simulink model "three_phase_diode_rectifier_updated"  (R2025a)
settings: Solver=VariableStepAuto  StartTime=0.0  StopTime=0.5  RelTol=1e-3
libraries: spsDiodeLib x6, spsACVoltageSourceLib x3, spsCurrentMeasurementLib x3, spsVoltageMeasurementLib x3, spsSeriesRLCBranchLib x2, spsMeanLib x1, spsTHDLib x1, spspowerguiLib x1
settings Model: Creator=yiğit  LastModifiedBy=yiğit

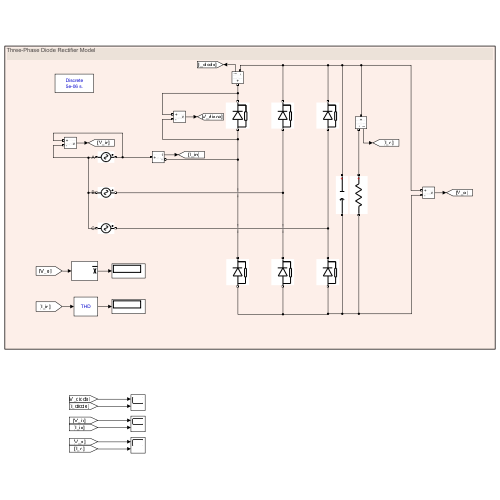
[thumbnail: Simulink's stored preview of the top-level diagram]
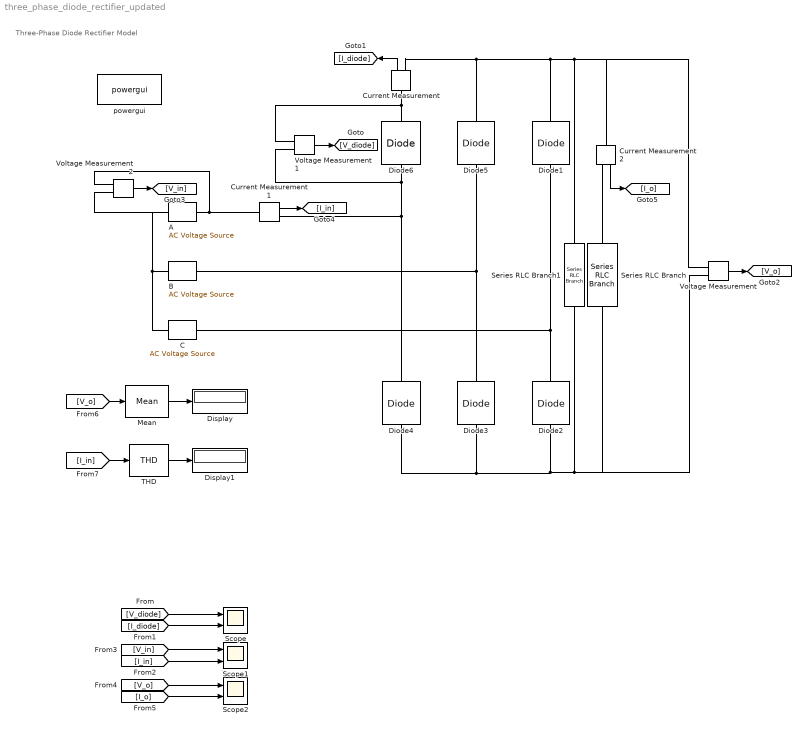
== system three_phase_diode_rectifier_updated ==
  note: Three-Phase Diode Rectifier Model
  A : spsACVoltageSourceLib/AC Voltage Source  Amplitude=136.082  Phase=0  Frequency=50  SampleTime=0  Measurements=None  BusType=swing  Pref=10e3  Qref=0  Qmin=-inf  Qmax=+inf
  B : spsACVoltageSourceLib/AC Voltage Source  Amplitude=136.082  Phase=120  Frequency=50  SampleTime=0  Measurements=None  BusType=swing  Pref=10e3  Qref=0  Qmin=-inf  Qmax=+inf
  C : spsACVoltageSourceLib/AC Voltage Source  Amplitude=136.082  Phase=240  Frequency=50  SampleTime=0  Measurements=None  BusType=swing  Pref=10e3  Qref=0  Qmin=-inf  Qmax=+inf
  Current Measurement : spsCurrentMeasurementLib/Current Measurement  PhasorSimulation=off  OutputType=Complex  PSBequivalent=0
  Current Measurement1 : spsCurrentMeasurementLib/Current Measurement  PhasorSimulation=off  OutputType=Complex  PSBequivalent=0
  Current Measurement2 : spsCurrentMeasurementLib/Current Measurement  PhasorSimulation=off  OutputType=Complex  PSBequivalent=0
  Diode{1..6} (6 alike) : spsDiodeLib/Diode  Ron=1e-3  Lon=0  Vf=0  IC=0  UseSnubber=0  Rs=1e6  Cs=1e-12  Measurements=off
  Display : Display
  Display1 : Display
  Mean : spsMeanLib/Mean  Freq=50  Vinit=0  Ts=0
  Scope : Scope  NumInputPorts=2
      settings: ActiveDisplayYMinimum=-34.164994069394211  ActiveDisplayYMaximum=260.46816184047532
  Scope1 : Scope  NumInputPorts=2
      settings: ActiveDisplayYMinimum=-170.10249999999996  ActiveDisplayYMaximum=170.10249999999996
  Scope2 : Scope  NumInputPorts=2
      settings: ActiveDisplayYMinimum=175.237742445763  ActiveDisplayYMaximum=464.02263493938636  DataLoggingVariableName=ScopeData2
  Series RLC Branch : spsSeriesRLCBranchLib/Series RLC Branch  LConnTagsString=__new0  RConnTagsString=__new0  BranchType=R  Resistance=25  Inductance=1e-3  SetiL0=off  InitialCurrent=0  Capacitance=1e-6  Setx0=off  InitialVoltage=0  Measurements=None
  Series RLC Branch1 : spsSeriesRLCBranchLib/Series RLC Branch  LConnTagsString=__new0  RConnTagsString=__new0  BranchType=C  Resistance=1  Inductance=1e-3  SetiL0=off  InitialCurrent=0  Capacitance=100e-6  Setx0=off  InitialVoltage=0  Measurements=None
  THD : spsTHDLib/THD  Freq=60  Ts=0
  Voltage Measurement : spsVoltageMeasurementLib/Voltage Measurement  PhasorSimulation=off  OutputType=Complex  PSBequivalent=0
  Voltage Measurement1 : spsVoltageMeasurementLib/Voltage Measurement  PhasorSimulation=off  OutputType=Complex  PSBequivalent=0
  Voltage Measurement2 : spsVoltageMeasurementLib/Voltage Measurement  PhasorSimulation=off  OutputType=Complex  PSBequivalent=0
  powergui : spspowerguiLib/powergui  Priority=1  SimulationMode=Discrete  SampleTime=5e-6  frequency=60  Iterations=50  frequencyindice=50  Pbase=100e6  ErrMax=1e-4  UnitsV=kV  UnitsW=MW  buscounter=0  FunctionMessages=off  echomessages=off  EnableUseOfTLC=off  CurrentSourceSwitches=off  DisableSnubberDevices=off  DisableRonSwitches=off  DisableVfSwitches=off  DisplayEquations=off  AutomaticDiscreteSolvers=off  SolverType=Tustin/Backward Euler (TBE)  Interpol=off  ExternalGateDelay=off  methode=off  Ts=100  x0status=blocks  SPID=on  SwTol=0  HookPort=off  NonlinearTolerance=1e-4  nMaxIteration=100  ContinueOnMaxIteration=off  RestoreLinks=warning  ResistiveCurrentMeasurement=off  Frange=[0:2:500]  Ylog=off  Xlog=on  ShowGrid=off  save=off  variable=ZData  structure=0  ZoomFFT=off  StartTime=0.0  cycles=1  DisplayStyle=1  fundamental=60  FreqAxis=off  MaxFrequency=1000  frequencyindicesteady=1  RmsSteady=1  display=off
  wires:
  Voltage Measurement1/1 -> [V_diode]
  Current Measurement/1 -> [I_diode]
  Voltage Measurement/1 -> [V_o]
  Voltage Measurement2/1 -> [V_in]
  Current Measurement1/1 -> [I_in]
  Current Measurement2/1 -> [I_o]
  [V_diode] -> Scope/1
  [I_diode] -> Scope/2
  [V_in] -> Scope1/1
  [I_in] -> Scope1/2
  [V_o] -> Scope2/1
  [I_o] -> Scope2/2
  [V_o] -> Mean/1
  Mean/1 -> Display/1
  [I_in] -> THD/1
  THD/1 -> Display1/1
  connections:
  C/LConn1 -- Voltage Measurement2/LConn2 -- A/LConn1 -- B/LConn1
  Diode4/RConn1 -- Diode6/LConn1 -- Voltage Measurement1/LConn2 -- Current Measurement1/RConn1
  Diode5/RConn1 -- Current Measurement2/LConn1 -- Voltage Measurement/LConn1 -- Series RLC Branch1/LConn1 -- Diode1/RConn1 -- Current Measurement/RConn1
  B/RConn1 -- Diode3/RConn1 -- Diode5/LConn1
  C/RConn1 -- Diode2/RConn1 -- Diode1/LConn1
  Diode4/LConn1 -- Diode3/LConn1 -- Series RLC Branch/RConn1 -- Voltage Measurement/LConn2 -- Series RLC Branch1/RConn1 -- Diode2/LConn1
  Diode6/RConn1 -- Current Measurement/LConn1 -- Voltage Measurement1/LConn1
  A/RConn1 -- Voltage Measurement2/LConn1 -- Current Measurement1/LConn1
  Current Measurement2/RConn1 -- Series RLC Branch/LConn1
